simulink model "ex_direct_lookup_table_4d_table_is_not_input"  (R2017b)
settings: Solver=FixedStepDiscrete  StartTime=0.0  StopTime=10.0  FixedStep=0.100000  RelTol=1e-3  EnableMultiTasking=on
PreLoadFcn:
  | a = reshape(1:2800, [4 5 20 7]);
settings Model: Creator=The MathWorks, Inc.  LastModifiedBy=hbourbou
settings DataIOCC: LimitDataPoints=on
settings OptimizationCC: ExpressionDepthLimit=2147483647  LifeSpan=inf
settings DebuggingCC: UnderspecifiedInitializationDetection=Classic  MergeDetectMultiDrivingBlocksExec=none  SolverPrmCheckMsg=warning  FcnCallInpInsideContextMsg=warning  StateNameClashWarn=warning  StrictBusMsg=Warning  SFUnexpectedBacktrackingDiag=warning  SFNoUnconditionalDefaultTransitionDiag=warning  SFExecutionAtInitializationDiag=none
settings HardwareCC: ProdBitPerPointer=32  ProdBitPerSizeT=32  ProdBitPerPtrDiffT=32  ProdLargestAtomicFloat=None  ProdIntDivRoundTo=Undefined  ProdEndianess=Unspecified  ProdWordSize=32  ProdHWDeviceType=32-bit Generic
settings ModelReferenceCC: PropagateSignalLabelsOutOfModel=off
settings RTWCC: Description=Generic Real-Time Target
settings CodeAppCC: StateflowObjectComments=on
settings GRTTargetCC: TargetLangStandard=C89/C90 (ANSI)  GeneratePreprocessorConditionals=Disable all  CombineOutputUpdateFcns=off  GRTInterface=on
settings ConfigComp: CovMetricSettings=dw  CovHtmlReporting=on  CovSaveCumulativeToWorkspaceVar=on  CovSaveSingleToWorkspaceVar=on  CovExternalEMLEnable=off

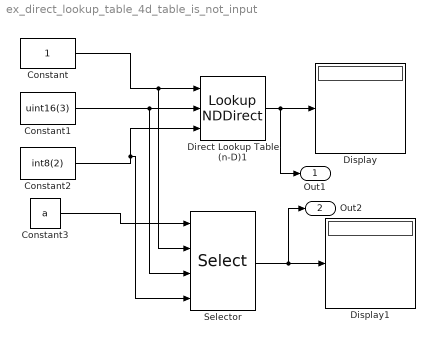
== system ex_direct_lookup_table_4d_table_is_not_input ==
  Constant : Constant
  Constant1 : Constant  Value=uint16(3)
  Constant2 : Constant  Value=int8(2)
  Constant3 : Constant  Value=a
  Direct Lookup Table (n-D)1 : LookupNDDirect  NumberOfTableDimensions=4  InputsSelectThisObjectFromTable=Column  Table=a
  Display : Display
  Display1 : Display
  Selector : Selector  NumberOfDimensions=4  IndexMode=Zero-based  InputPortWidth=3  IndexOptions=Select all,Index vector (port),Index vector (port),Index vector (port)  Indices=[1 3],1,1,1  OutputSizes=1,1,1,1
  Out1 : Outport
  Out2 : Outport  Port=2
  wires:
  Constant/1 -> Direct Lookup Table (n-D)1/1, Selector/2
  Constant1/1 -> Direct Lookup Table (n-D)1/2, Selector/3
  Constant2/1 -> Direct Lookup Table (n-D)1/3, Selector/4
  Constant3/1 -> Selector/1
  Selector/1 -> Out2/1, Display1/1
  Direct Lookup Table (n-D)1/1 -> Out1/1, Display/1
